simulink model "C_to_F_converter"  (R2015a)
settings: Solver=ode45  StartTime=0.0  StopTime=10.0  RelTol=1e-3
settings Model: Creator=pc  LastModifiedBy=pc

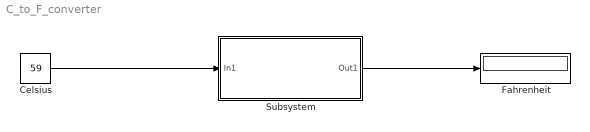
== system C_to_F_converter ==
  Celsius : Constant  Value=59
  Fahrenheit : Display
  Subsystem : Subsystem
  wires:
  Celsius/1 -> Subsystem/1(In1)
  Subsystem/1(Out1) -> Fahrenheit/1

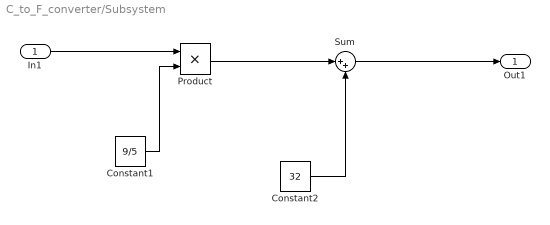
== system C_to_F_converter/Subsystem ==
  In1 : Inport
  Constant1 : Constant  Value=9/5
  Constant2 : Constant  Value=32
  Product : Product
  Sum : Sum  Inputs=|++
  Out1 : Outport
  wires:
  Constant2/1 -> Sum/2
  Sum/1 -> Out1/1
  In1/1 -> Product/1
  Constant1/1 -> Product/2
  Product/1 -> Sum/1
